simulink model "PMSM_FOC_Traction"  (R2020b)
settings: Solver=FixedStepAuto  StartTime=0.0  StopTime=10  RelTol=1e-3
model workspace (MAT data in the model file):
  wc : Simulink.Parameter (value not decoded)
values from neighbouring files (symbols this model uses):
  CL_Param = tmp_CL_Param    [PMSM_Parameters.m]
  Cosine_table = [1,0.999995293095708,0.999990587122738,0.999985881149769,0.999981174245477,0.999967055395246,0.999952936545014,0.999938818626106,0.999924698844552,0.999901168979704,0.999877639114857,0.999854108318687,0.999830577522516,0.999797635711730,0.999764694832265,0.999731753021479,0.999698810279369,0.999656459316611,0.999614108353853,0.999571758322418,0.999529405497015,0.999477646313608,0.999425887130201,0 ...(+75635 chars)    [Motor_Table.m]
  ctrlParamsPI = tmp_ctrlParamsPI    [PMSM_Parameters.m]
  Flux_weak = tmp_Fluxweak_struct    [PMSM_Parameters.m]
  FluxObsever = tmp_FluxObsever_struct    [PMSM_Parameters.m]
  Hall_Parameter = tmp_Hall_struct    [PMSM_Parameters.m]
  HFI = tmp_HFI_struct    [PMSM_Parameters.m]
  inverter = struct    [PMSM_Parameters.m]
  MTPA_id_table = [-1.39452500000000,-1.36697494250000,-1.33970177000000,-1.31270548250000,-1.28598608000000,-1.25954356250000,-1.23337793000000,-1.20748918250000,-1.18187732000000,-1.15654234250000,-1.13148425000000,-1.10670304250000,-1.08219872000000,-1.05797128250000,-1.03402073000000,-1.01034706250000,-0.986950280000000,-0.963830382500000,-0.940987370000000,-0.918421242500000,-0.896132000000000,-0.8741196425000 ...(+3439 chars)    [Motor_Table.m]
  MTPA_iq_table = [-10.2740250000000,-10.1791705677750,-10.0840783722000,-9.98875081492500,-9.89319029760000,-9.79739922187500,-9.70137998940000,-9.60513500182500,-9.50866666080000,-9.41197736797500,-9.31506952500000,-9.21794553352500,-9.12060779520000,-9.02305871167500,-8.92530068460000,-8.82733611562500,-8.72916740640000,-8.63079695857500,-8.53222717380000,-8.43346045372500,-8.33449920000000,-8.23534581427500,-8. ...(+3121 chars)    [Motor_Table.m]
  MTPA_Te_Max = single(1.50)    [Motor_Table.m]
  MTPA_Te_Min = single(-1.50)    [Motor_Table.m]
  OPL_Param = tmp_OPL_Param    [PMSM_Parameters.m]
  pmsm = struct    [PMSM_Parameters.m]
  Resolver_Parameter = tmp_Resolver_struct    [PMSM_Parameters.m]
  Sine_table = [0,0.00153398793190718,0.00306797679513693,0.00460196565836668,0.00613595545291901,0.00766988657414913,0.00920381769537926,0.0107377488166094,0.0122716808691621,0.0138054965063930,0.0153393121436238,0.0168731296434999,0.0184069443494082,0.0199405867606401,0.0214742291718721,0.0230078706517816,0.0245415139943361,0.0260749254375696,0.0276083368808031,0.0291417483240366,0.0306751597672701,0.032208281 ...(+75648 chars)    [Motor_Table.m]
  SMO = temp_SMO    [PMSM_Parameters.m]
undefined symbols (not defined in the file or in its folder): DiscIntNeverNeededParam, Kiv, Kiw, Kpv, Kpw, magnitude, sigbuilder_block, SVPWM, Vdc
libraries: powerlib x29, fl_lib x18, simulink x7, nesl_utility x7, pid_lib x5, dspstat3 x4, eeGeneralControl x4, eeDiscretePi x2, powerlib_extras x1, ee_lib x1
(part 2 of 6)

== system PMSM_FOC_Traction/PMSM/Resolver_Angle_cacl ==
  Vp_Vx_Vy : Inport
  2*pi : Constant  Value=2*pi  OutDataTypeStr=single  SampleTime=-1
  A : Selector  IndexMode=Zero-based  InputPortWidth=3  IndexOptions=Index vector (dialog)  Indices=0  OutputSizes=1
  B : Selector  IndexMode=Zero-based  InputPortWidth=3  IndexOptions=Index vector (dialog)  Indices=1  OutputSizes=1
  C : Selector  IndexMode=Zero-based  InputPortWidth=3  IndexOptions=Index vector (dialog)  Indices=2  OutputSizes=1
  Constant : Constant  Value=pmsm.PolePairs  OutDataTypeStr=single  SampleTime=-1
  Discrete-Time Integrator : DiscreteIntegrator  SampleTime=-1  ICPrevOutput=DiscIntNeverNeededParam  ICPrevScaledInput=DiscIntNeverNeededParam
  Gain : Gain  Gain=60/(2*pi)
  Math Function : Math  Operator=mod  SignedPower=on  SaturateOnIntegerOverflow=on
  PID Controller : pid_lib/PID Controller  Controller=PI  Form=Parallel  TimeDomain=Discrete-time  UseExternalTs=off  SampleTime=-1  IntegratorMethod=Forward Euler  FilterMethod=Forward Euler  ControllerParametersSource=internal  P=15  I=2.5e5  D=0  UseFilter=off  N=100  TunerSelectOption=Transfer Function Based (PID Tuner App)  InitialConditionSource=internal  InitialConditionForIntegrator=0  InitialConditionForFilter=0  DifferentiatorICPrevScaledInput=0  ExternalReset=none  TrackingMode=off  Kt=1  LimitOutput=off  SatLimitsSource=internal  UpperSaturationLimit=inf  LowerSaturationLimit=-inf  LinearizeAsGain=on  AntiWindupMode=none  Kb=1  POutMin=[]  POutMax=[]  IOutMin=[]  IOutMax=[]  DOutMin=[]  DOutMax=[]  NOutMin=[]  NOutMax=[]  SumOutMin=[]  SumOutMax=[]  SaturationOutMin=[]  SaturationOutMax=[]  PParamMin=[]  PParamMax=[]  IParamMin=[]  IParamMax=[]  DParamMin=[]  DParamMax=[]  NParamMin=[]  NParamMax=[]  KbParamMin=[]  KbParamMax=[]  KtParamMin=[]  KtParamMax=[]  KbOutMin=[]  KbOutMax=[]  KtOutMin=[]  KtOutMax=[]  IntegratorOutMin=[]  IntegratorOutMax=[]  FilterOutMin=[]  FilterOutMax=[]  SumI1OutMin=[]  SumI1OutMax=[]  SumI2OutMin=[]  SumI2OutMax=[]  SumI3OutMin=[]  SumI3OutMax=[]  SumI4OutMin=[]  SumI4OutMax=[]  SumDOutMin=[]  SumDOutMax=[]  DifferentiatorOutMin=[]  DifferentiatorOutMax=[]  FilterDiffOutCoefMin=[]  FilterDiffOutCoefMax=[]  ReciprocalOutMin=[]  ReciprocalOutMax=[]  SumDenOutMin=[]  SumDenOutMax=[]  SumNumOutMin=[]  SumNumOutMax=[]  DivideOutMin=[]  DivideOutMax=[]  UdiffTsProdOutMin=[]  UdiffTsProdOutMax=[]  NTsProdOutMin=[]  NTsProdOutMax=[]  UintegralTsProdOutMin=[]  UintegralTsProdOutMax=[]  UngainTsProdOutMin=[]  UngainTsProdOutMax=[]  IntegratorContinuousStateAttributes=''  IntegratorStateMustResolveToSignalObject=off  IntegratorRTWStateStorageClass=Auto  FilterContinuousStateAttributes=''  FilterStateMustResolveToSignalObject=off  FilterRTWStateStorageClass=Auto  ParallelPVariant=InternalParameters  IdealPVariant=Disabled  IVariant=InternalParameters  DVariant=Disabled  IntegratorVariant=Discrete  SatVariant=Disabled  AWVariant=Passthrough  PCopyVariant=Disabled  TRVariant=Disabled  FdbkBlocksVariant=Forward  IdealPFdbkVariant=Disabled  SatFdbkVariant=Disabled  DerivativeFilterVariant=Disabled  NVariant=Disabled  NCopyVariant=Disabled_SignalSpec  FilterICVariant=Disabled  IntegratorICVariant=InternalICs  ExternalResetVariant=Disabled  TRSumVariant=Passthrough  SumFdbkVariant=Disabled  SumVariant=Sum_PI  TsampFilterVariant=InternalTs  TsampNgainVariant=Passthrough  TsampIntegralVariant=Passthrough  ExternalSaturationOutDataTypeStr=Inherit: Same as second input
  Product : Product  OutDataTypeStr=single
  Product{1..4} (4 alike) : Product
  Quantizer : Quantizer  QuantizationInterval=1e-5
  Quantizer1 : Quantizer  QuantizationInterval=1e-5
  Quantizer2 : Quantizer  QuantizationInterval=1e-5
  Scope : Scope  NumInputPorts=2
  Scope{1,3..4,6} (4 alike) : Scope
  Scope2 : Scope  NumInputPorts=2
  Scope5 : Scope  NumInputPorts=2
  Sum1 : Sum  Inputs=-+
  Trigonometric Function : Trigonometry  Operator=sincos
  Unit Delay4 : UnitDelay  SampleTime=-1  HasFrameUpgradeWarning=on
  "pole pairs " : Gain  Gain=pmsm.PolePairs  OutDataTypeStr=single
  Velocity : Outport  VectorParamsAs1DForOutWhenUnconnected=off
  Angle : Outport  Port=2  VectorParamsAs1DForOutWhenUnconnected=off
  wires:
  Quantizer/1 -> Scope1/1, Product3/1
  Quantizer1/1 -> Product4/2
  Product2/1 -> Scope2/2, Product4/1
  Product4/1 -> Scope/2, Sum1/2
  Trigonometric Function/2 -> Product2/2
  Vp_Vx_Vy/1 -> C/1, B/1, A/1
  Unit Delay4/1 -> Product/2
  Sum1/1 -> PID Controller/1
  Product3/1 -> Scope/1, Sum1/1
  Constant/1 -> Product/1
  Quantizer2/1 -> Product2/1, Product1/1
  Product/1 -> Trigonometric Function/1
  Trigonometric Function/1 -> Product1/2
  Product1/1 -> Scope2/1, Product3/2
  Math Function/1 -> Angle/1, Scope4/1  "Angle1"
  Gain/1 -> Velocity/1, Scope3/1  "Speed1"
  Discrete-Time Integrator/1 -> Scope6/1, "pole pairs "/1, Unit Delay4/1
  "pole pairs "/1 -> Math Function/1
  PID Controller/1 -> Discrete-Time Integrator/1, Gain/1
  2*pi/1 -> Math Function/2
  A/1 -> Quantizer2/1  "Vp"
  B/1 -> Scope5/1, Quantizer/1, Scope5/2  "Vx"
  C/1 -> Quantizer1/1  "Vy"

== system PMSM_FOC_Traction/PMSM/Resolver_Angle_cacl1 ==
  Vp_Vx_Vy : Inport
  2*pi : Constant  Value=2*pi  OutDataTypeStr=single  SampleTime=-1
  A : Selector  IndexMode=Zero-based  InputPortWidth=3  IndexOptions=Index vector (dialog)  Indices=0  OutputSizes=1
  B : Selector  IndexMode=Zero-based  InputPortWidth=3  IndexOptions=Index vector (dialog)  Indices=1  OutputSizes=1
  C : Selector  IndexMode=Zero-based  InputPortWidth=3  IndexOptions=Index vector (dialog)  Indices=2  OutputSizes=1
  Constant : Constant  Value=pmsm.PolePairs  OutDataTypeStr=single  SampleTime=-1
  Discrete-Time Integrator : DiscreteIntegrator  SampleTime=-1  ICPrevOutput=DiscIntNeverNeededParam  ICPrevScaledInput=DiscIntNeverNeededParam
  Gain : Gain  Gain=60/(2*pi)
  LPF : DiscreteFilter  Numerator=[0 0.04]  Denominator=[1 -0.96]  SampleTime=inverter.Ts
  Math Function : Math  Operator=mod  SignedPower=on  SaturateOnIntegerOverflow=on
  PID Controller : pid_lib/PID Controller  Controller=PI  Form=Parallel  TimeDomain=Discrete-time  UseExternalTs=off  SampleTime=-1  IntegratorMethod=Forward Euler  FilterMethod=Forward Euler  ControllerParametersSource=internal  P=120  I=2500  D=0  UseFilter=off  N=100  TunerSelectOption=Transfer Function Based (PID Tuner App)  InitialConditionSource=internal  InitialConditionForIntegrator=0  InitialConditionForFilter=0  DifferentiatorICPrevScaledInput=0  ExternalReset=none  TrackingMode=off  Kt=1  LimitOutput=off  SatLimitsSource=internal  UpperSaturationLimit=inf  LowerSaturationLimit=-inf  LinearizeAsGain=on  AntiWindupMode=none  Kb=1  POutMin=[]  POutMax=[]  IOutMin=[]  IOutMax=[]  DOutMin=[]  DOutMax=[]  NOutMin=[]  NOutMax=[]  SumOutMin=[]  SumOutMax=[]  SaturationOutMin=[]  SaturationOutMax=[]  PParamMin=[]  PParamMax=[]  IParamMin=[]  IParamMax=[]  DParamMin=[]  DParamMax=[]  NParamMin=[]  NParamMax=[]  KbParamMin=[]  KbParamMax=[]  KtParamMin=[]  KtParamMax=[]  KbOutMin=[]  KbOutMax=[]  KtOutMin=[]  KtOutMax=[]  IntegratorOutMin=[]  IntegratorOutMax=[]  FilterOutMin=[]  FilterOutMax=[]  SumI1OutMin=[]  SumI1OutMax=[]  SumI2OutMin=[]  SumI2OutMax=[]  SumI3OutMin=[]  SumI3OutMax=[]  SumI4OutMin=[]  SumI4OutMax=[]  SumDOutMin=[]  SumDOutMax=[]  DifferentiatorOutMin=[]  DifferentiatorOutMax=[]  FilterDiffOutCoefMin=[]  FilterDiffOutCoefMax=[]  ReciprocalOutMin=[]  ReciprocalOutMax=[]  SumDenOutMin=[]  SumDenOutMax=[]  SumNumOutMin=[]  SumNumOutMax=[]  DivideOutMin=[]  DivideOutMax=[]  UdiffTsProdOutMin=[]  UdiffTsProdOutMax=[]  NTsProdOutMin=[]  NTsProdOutMax=[]  UintegralTsProdOutMin=[]  UintegralTsProdOutMax=[]  UngainTsProdOutMin=[]  UngainTsProdOutMax=[]  IntegratorContinuousStateAttributes=''  IntegratorStateMustResolveToSignalObject=off  IntegratorRTWStateStorageClass=Auto  FilterContinuousStateAttributes=''  FilterStateMustResolveToSignalObject=off  FilterRTWStateStorageClass=Auto  ParallelPVariant=InternalParameters  IdealPVariant=Disabled  IVariant=InternalParameters  DVariant=Disabled  IntegratorVariant=Discrete  SatVariant=Disabled  AWVariant=Passthrough  PCopyVariant=Disabled  TRVariant=Disabled  FdbkBlocksVariant=Forward  IdealPFdbkVariant=Disabled  SatFdbkVariant=Disabled  DerivativeFilterVariant=Disabled  NVariant=Disabled  NCopyVariant=Disabled_SignalSpec  FilterICVariant=Disabled  IntegratorICVariant=InternalICs  ExternalResetVariant=Disabled  TRSumVariant=Passthrough  SumFdbkVariant=Disabled  SumVariant=Sum_PI  TsampFilterVariant=InternalTs  TsampNgainVariant=Passthrough  TsampIntegralVariant=Passthrough  ExternalSaturationOutDataTypeStr=Inherit: Same as second input
  Product : Product  OutDataTypeStr=single
  Product{1..4} (4 alike) : Product
  Quantizer : Quantizer  QuantizationInterval=1e-5
  Quantizer1 : Quantizer  QuantizationInterval=1e-5
  Quantizer2 : Quantizer  QuantizationInterval=1e-5
  Scope : Scope  NumInputPorts=2
  Scope{1,3..4,6} (4 alike) : Scope
  Scope2 : Scope  NumInputPorts=2
  Scope5 : Scope  NumInputPorts=2
  Sum1 : Sum  Inputs=-+
  Trigonometric Function : Trigonometry  Operator=sincos
  Unit Delay4 : UnitDelay  SampleTime=-1  HasFrameUpgradeWarning=on
  "pole pairs " : Gain  Gain=pmsm.PolePairs  OutDataTypeStr=single
  Velocity : Outport  VectorParamsAs1DForOutWhenUnconnected=off
  Angle : Outport  Port=2  VectorParamsAs1DForOutWhenUnconnected=off
  wires:
  Quantizer/1 -> Scope1/1, Product3/1, Scope5/2
  Quantizer1/1 -> Product4/2
  Product2/1 -> Scope2/2, Product4/1
  Product4/1 -> Scope/2, Sum1/2
  Trigonometric Function/2 -> Product2/2
  Vp_Vx_Vy/1 -> C/1, B/1, A/1
  Unit Delay4/1 -> Product/2
  Sum1/1 -> PID Controller/1
  Product3/1 -> Scope/1, Sum1/1
  Constant/1 -> Product/1
  Quantizer2/1 -> Product2/1, Product1/1
  Product/1 -> Trigonometric Function/1
  Trigonometric Function/1 -> Product1/2
  Product1/1 -> Scope2/1, Product3/2
  Math Function/1 -> Angle/1, Scope4/1  "Angle"
  Gain/1 -> LPF/1, Scope3/1  "Speed"
  Discrete-Time Integrator/1 -> Scope6/1, "pole pairs "/1, Unit Delay4/1
  "pole pairs "/1 -> Math Function/1
  PID Controller/1 -> Discrete-Time Integrator/1, Gain/1
  2*pi/1 -> Math Function/2
  A/1 -> Quantizer2/1  "Vp"
  B/1 -> Scope5/1, Quantizer/1  "Vx"
  C/1 -> Quantizer1/1  "Vy"
  LPF/1 -> Velocity/1

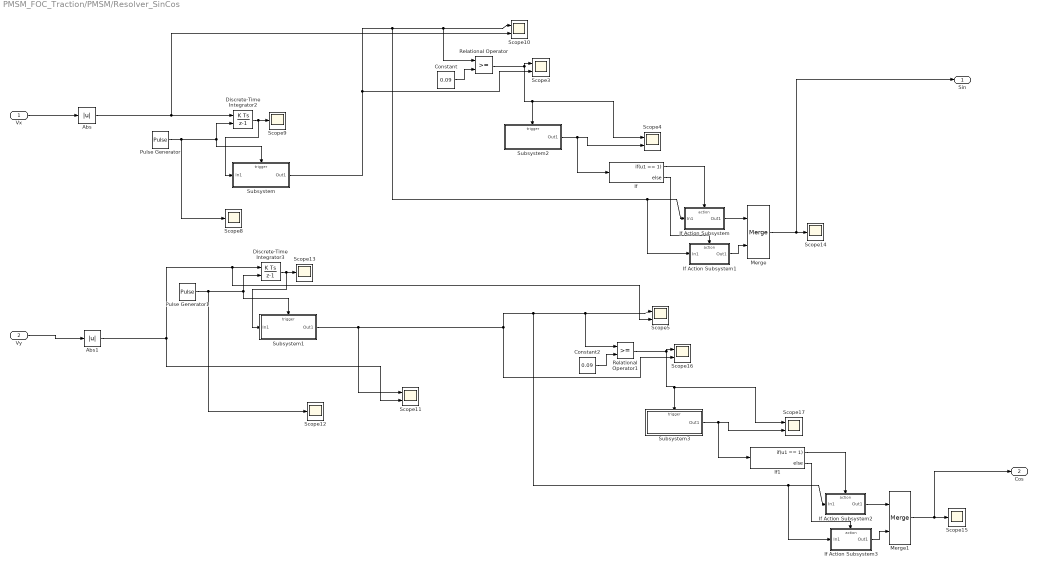
== system PMSM_FOC_Traction/PMSM/Resolver_SinCos ==
  Vx : Inport
  Vy : Inport  Port=2
  Abs : Abs
  Abs1 : Abs
  Constant : Constant  Value=0.09
  Constant2 : Constant  Value=0.09
  Discrete-Time Integrator2 : DiscreteIntegrator  gainval=15625  ExternalReset=falling  SampleTime=-1  ICPrevOutput=DiscIntNeverNeededParam  ICPrevScaledInput=DiscIntNeverNeededParam
  Discrete-Time Integrator3 : DiscreteIntegrator  gainval=15625  ExternalReset=falling  SampleTime=-1  ICPrevOutput=DiscIntNeverNeededParam  ICPrevScaledInput=DiscIntNeverNeededParam
  If : If  IfExpression=u1 == 1
  If Action Subsystem : Subsystem  TreatAsAtomicUnit=on
  If Action Subsystem1 : Subsystem  TreatAsAtomicUnit=on
  If Action Subsystem2 : Subsystem  TreatAsAtomicUnit=on
  If Action Subsystem3 : Subsystem  TreatAsAtomicUnit=on
  If1 : If  IfExpression=u1 == 1
  Merge : Merge
  Merge1 : Merge
  Pulse Generator : DiscretePulseGenerator  PulseType=Time based  Period=inverter.Ts  PulseWidth=5
  Pulse Generator1 : DiscretePulseGenerator  PulseType=Time based  Period=inverter.Ts  PulseWidth=5
  Relational Operator : RelationalOperator  OutDataTypeStr=boolean  RndMeth=Simplest
  Relational Operator1 : RelationalOperator  OutDataTypeStr=boolean  RndMeth=Simplest
  Scope{3..5,10..11,16..17} (7 alike) : Scope  NumInputPorts=2
  Scope{8..9,12..15} (6 alike) : Scope
  Subsystem : Subsystem
  Subsystem1 : Subsystem
  Subsystem2 : Subsystem
  Subsystem3 : Subsystem
  Sin : Outport
  Cos : Outport  Port=2
  wires:
  Discrete-Time Integrator2/1 -> Subsystem/1(In1), Scope9/1
  Subsystem/1(Out1) -> If Action Subsystem1/1(In1), If Action Subsystem/1(In1), Relational Operator/1, Scope10/1, Scope3/2
  Subsystem2/1(Out1) -> If/1, Scope4/2
  Pulse Generator/1 -> Scope8/1, Discrete-Time Integrator2/2, Subsystem/Trigger
  If Action Subsystem2/1(Out1) -> Merge1/1
  If1/1 -> If Action Subsystem2/Action
  Relational Operator1/1 -> Scope17/1, Subsystem3/Trigger, Scope16/1
  Merge1/1 -> Cos/1, Scope15/1
  Constant2/1 -> Relational Operator1/2
  Subsystem3/1(Out1) -> If1/1, Scope17/2
  Abs1/1 -> Scope5/2, Discrete-Time Integrator3/1, Scope11/2
  If/2 -> If Action Subsystem1/Action
  Constant/1 -> Relational Operator/2
  If1/2 -> If Action Subsystem3/Action
  Relational Operator/1 -> Scope4/1, Subsystem2/Trigger, Scope3/1
  Pulse Generator1/1 -> Scope12/1, Discrete-Time Integrator3/2, Subsystem1/Trigger
  Abs/1 -> Scope10/2, Discrete-Time Integrator2/1
  Discrete-Time Integrator3/1 -> Subsystem1/1(In1), Scope13/1
  Merge/1 -> Sin/1, Scope14/1
  If Action Subsystem1/1(Out1) -> Merge/2
  Subsystem1/1(Out1) -> If Action Subsystem3/1(In1), If Action Subsystem2/1(In1), Relational Operator1/1, Scope5/1, Scope16/2, Scope11/1
  If Action Subsystem/1(Out1) -> Merge/1
  If Action Subsystem3/1(Out1) -> Merge1/2
  If/1 -> If Action Subsystem/Action
  Vx/1 -> Abs/1
  Vy/1 -> Abs1/1

== system PMSM_FOC_Traction/PMSM/SVPWM2 ==
  Gate : Inport
  Duty : Inport  Port=2
  Add{1..6} (6 alike) : Sum  Inputs=+-
  Bus Creator : BusCreator  Inputs=6
  Demux1 : Demux  Outputs=6
  Gain2 : Gain  Gain=4200
  Product{1..6} (6 alike) : Product
  Relay{,1..5} (6 alike) : Relay  OnOutputValue=0  OffOutputValue=1
  Repeating Sequence2 : simulink/Sources/Repeating Sequence  rep_seq_t=[0 inverter.Ts/2 inverter.Ts]  rep_seq_y=[0 4200 0]
  Scope : Scope  NumInputPorts=2
  Scope1 : Scope  NumInputPorts=2
  pulse : Outport
  wires:
  Repeating Sequence2/1 -> Add1/1, Add4/1, Add2/1, Add5/1, Add6/1, Add3/1
  Product2/1 -> Add2/2
  Product3/1 -> Add3/2
  Add3/1 -> Relay2/1
  Add2/1 -> Relay1/1
  Add1/1 -> Relay/1
  Product1/1 -> Add1/2
  Bus Creator/1 -> pulse/1
  Gate/1 -> Demux1/1
  Demux1/1 -> Product1/1, Scope/1
  Demux1/3 -> Product2/1
  Demux1/5 -> Product3/1
  Gain2/1 -> Product4/2, Product1/2, Product5/2, Product6/2, Product3/2, Product2/2
  Demux1/2 -> Product4/1
  Demux1/4 -> Product5/1
  Demux1/6 -> Scope1/2, Product6/1
  Add4/1 -> Relay3/1
  Add5/1 -> Relay4/1
  Add6/1 -> Relay5/1
  Product6/1 -> Add6/2
  Product5/1 -> Add5/2
  Product4/1 -> Add4/2
  Relay/1 -> Scope/2, Bus Creator/1
  Relay3/1 -> Bus Creator/2
  Relay1/1 -> Bus Creator/3
  Relay2/1 -> Bus Creator/5
  Relay5/1 -> Bus Creator/6, Scope1/1
  Duty/1 -> Gain2/1
  Relay4/1 -> Bus Creator/4

== system PMSM_FOC_Traction/PMSM/SpeedAndAngle ==
  Hall : Inport
  Counter : Inport  Port=2
  ACC_OMG : Subsystem  TreatAsAtomicUnit=on
      settings: RTWSystemCode=Nonreusable function  RTWFcnNameOpts=Use subsystem name
  ADC_IRQ : Subsystem  TreatAsAtomicUnit=on
      settings: RTWSystemCode=Nonreusable function  RTWFcnNameOpts=Use subsystem name
  Demux : Demux  Outputs=3
  Scope : Scope
  Hall_Angle : Outport
  Hall_Speed_RPM : Outport  Port=2
  Six_theta : Outport  Port=3
  wires:
  Demux/2 -> ACC_OMG/3(HallB)
  Demux/3 -> ACC_OMG/4(HallC)
  ACC_OMG/1(Hall_SpeedRPM) -> Hall_Speed_RPM/1
  Counter/1 -> ACC_OMG/1(Timer_Counter), ADC_IRQ/1(Counter_ADC_IRQ)
  Demux/1 -> ACC_OMG/2(HallA)
  ACC_OMG/5(Six_theta) -> ADC_IRQ/5(Six_theta)
  ACC_OMG/2(Acc) -> ADC_IRQ/2(Acc)
  ACC_OMG/3(OMG) -> ADC_IRQ/3(OMG)
  Hall/1 -> ACC_OMG/Trigger, Demux/1
  ACC_OMG/4(Counter) -> ADC_IRQ/4(Counter_Hall_IRQ)
  ADC_IRQ/1(Hall_Angle) -> Hall_Angle/1, Scope/1
  ACC_OMG/6(Six_theta1) -> Six_theta/1

== system PMSM_FOC_Traction/PMSM/Timer_Counter ==
  Add2 : Sum
  Constant3 : Constant  OutDataTypeStr=single
  Memory : Memory  InheritSampleTime=on
  Counter : Outport
  wires:
  Add2/1 -> Counter/1, Memory/1
  Constant3/1 -> Add2/1
  Memory/1 -> Add2/2

== system PMSM_FOC_Traction/PMSM/Timer_Counter1 ==
  Add2 : Sum
  Constant3 : Constant  OutDataTypeStr=single
  Memory : Memory  InheritSampleTime=on
  Counter : Outport
  wires:
  Add2/1 -> Counter/1, Memory/1
  Constant3/1 -> Add2/1
  Memory/1 -> Add2/2

== system PMSM_FOC_Traction/PMSM/W_R ==
  w : Inport
  Angular Velocity Source : fl_lib/Mechanical/Mechanical Sources/Ideal Angular Velocity Source
  Mechanical Rotational Reference2 : fl_lib/Mechanical/Rotational Elements/Mechanical Rotational Reference
  Simulink-PS Converter : nesl_utility/Simulink-PS Converter  PhysicalDomain=network_engine_domain  SubClassName=ps_input  LeftPortType=input  RightPortType=output  PseudoPeriodic=off  Frequencies=[]  NoiseDistribution=none  NoiseParameters=[]  Unit=rad/s  AffineConversion=off  FilteringAndDerivatives=zero  SimscapeFilterOrder=1  InputFilterTimeConstant=0.0001  UdotUserProvided=1
  Torque Sensor : Subsystem
  R : PMIOPort  Side=Right
  C : PMIOPort  Port=2  Side=Right
  tag scope: wref=global
  wires:
  w/1 -> [wref], Simulink-PS Converter/1
  connections:
  Mechanical Rotational Reference2/LConn1 -- C/RConn1 -- Angular Velocity Source/RConn2
  Simulink-PS Converter/RConn1 -- Angular Velocity Source/RConn1
  Torque Sensor/LConn1 -- R/RConn1
  Torque Sensor/RConn1 -- Angular Velocity Source/LConn1

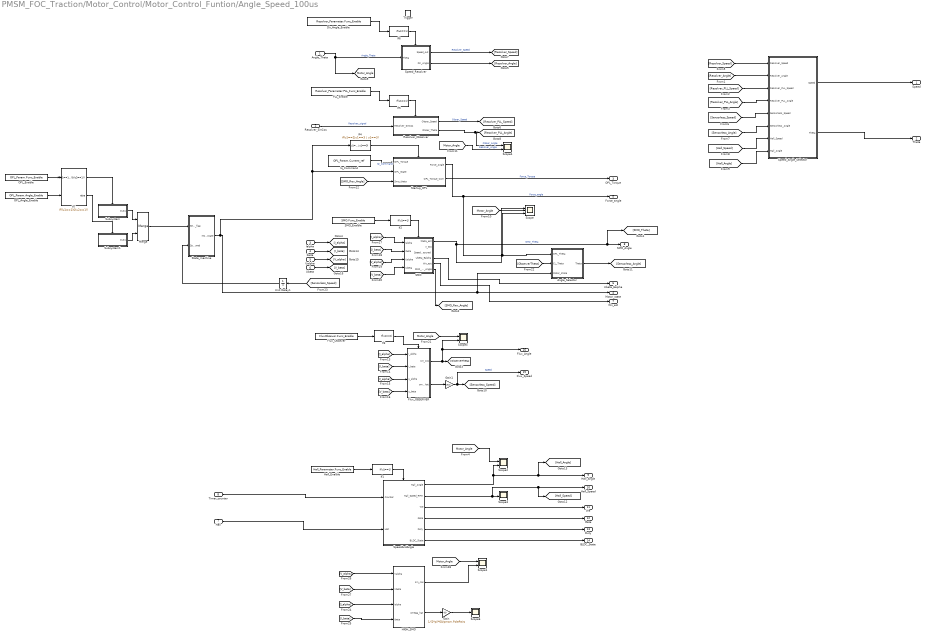
== system PMSM_FOC_Traction/Motor_Control/Motor_Control_Funtion/Angle_Speed_100us ==
  Angle_Theta : Inport  OutMin=0  OutMax=2*pi
  Resolver_SinCos : Inport  Port=2  OutMin=0  OutMax=2*pi
  Ialpha : Inport  Port=3
  Ibeta : Inport  Port=4
  Ualpha : Inport  Port=5
  Ubeta : Inport  Port=6
  Hall : Inport  Port=7
  Timer_counter : Inport  Port=8
  Trigger : TriggerPort  TriggerType=function-call  VariantControl=Variant  SampleTimeType=periodic  SampleTime=-1  PortDimensions=1
  Angle_Selector : Subsystem  TreatAsAtomicUnit=on
      settings: RTWSystemCode=Nonreusable function  RTWFcnNameOpts=Use subsystem name
  Dir_Angle_Enable : Constant  Value=Resolver_Parameter.Func_Enable  OutDataTypeStr=uint8
  Flux_OBSERVER : Subsystem
  Flux_Obsever : Constant  Value=FluxObsever.Func_Enable  OutDataTypeStr=uint8
  Gain : Gain  Gain=1/(2*pi)*60/pmsm.PolePairs
  Gain1 : Gain  Gain=15/pi  OutDataTypeStr=Inherit: Same as input  ParamDataTypeStr=Inherit: Same as input
  HIGH_SMO : Subsystem
      mask Display:
      | port_label('input',1,'U_\alpha','texmode','on');
      | port_label('input',2,'U_\beta','texmode','on');
      | port_label('input',3,'I_\alpha','texmode','on');
      | port_label('input',4,'I_\beta','texmode','on');
      | 
      | port_label('output',1,'sin(\theta_e)cos(\theta_e)','texmode','on');
      | port_label('output',2,'\omega_e','texmode','on');
      | 
      | fprintf('HSMO');
  Hall_Enalble : Constant  Value=Hall_Parameter.Func_Enable  OutDataTypeStr=uint8
  If{1..3,5..6} (5 alike) : If  IfExpression=u1==1  ShowElse=off
  If4 : If  IfExpression=u1==2|u1==3 | u1==3  ShowElse=off
  If7 : If  NumInputs=2  IfExpression=(u1==1)&(u2==1)
  Iq_Command : Constant  Value=OPL_Param.Current_ref  SampleTime=-1
  Merge : Merge
  OPL_Angle_Enable : Constant  Value=OPL_Param.Angle_Enable  OutDataTypeStr=uint8
  OPL_Enable : Constant  Value=OPL_Param.Func_Enable  OutDataTypeStr=uint8
  PLL_Enable : Constant  Value=Resolver_Parameter.PLL_Func_Enable  OutDataTypeStr=uint8
  Resolver_Observer : Subsystem
      settings: RTWSystemCode=Nonreusable function  RTWFcnNameOpts=Use subsystem name
  SMO : Subsystem  TreatAsAtomicUnit=on
      settings: RTWSystemCode=Nonreusable function  RTWFcnNameOpts=Use subsystem name
  SMO_Enalble : Constant  Value=SMO.Func_Enable  OutDataTypeStr=uint8
  Scope : Scope  NumInputPorts=3
  Scope{1..2,4..5} (4 alike) : Scope  NumInputPorts=2
  Scope3 : Scope
  Scope6 : Scope
  SpeedAndAngle : Subsystem
      settings: RTWSystemCode=Nonreusable function  RTWFcnNameOpts=Use subsystem name  RTWFileNameOpts=Use subsystem name
  Speed_Angle_Selector : Subsystem
  Speed_Resolver : Subsystem  TreatAsAtomicUnit=on
      settings: RTWSystemCode=Nonreusable function  RTWFcnNameOpts=Use subsystem name
  Startup_OPL : Subsystem  TreatAsAtomicUnit=on  SystemSampleTime=inverter.Ts
      settings: RTWSystemCode=Nonreusable function  RTWFcnNameOpts=Use subsystem name
  State_machine : Stateflow chart  TreatAsAtomicUnit=on
      settings: RTWSystemCode=Nonreusable function  RTWFcnNameOpts=Use subsystem name
  Subsystem : Subsystem
  Subsystem1 : Subsystem
  Unit Delay1 : UnitDelay  SampleTime=-1  HasFrameUpgradeWarning=on
  Speed : Outport
  Theta : Outport  Port=2
  OPL_Torque : Outport  Port=3
  Motor_state : Outport  Port=4
  Force_angle : Outport  Port=5
  Ubeta_Ealpha : Outport  Port=6
  Wn_est : Outport  Port=7
  SMO_Angle : Outport  Port=8
  Hall_Angle : Outport  Port=9
  Hall_Speed : Outport  Port=10
  We : Outport  Port=11
  Gate : Outport  Port=12  VectorParamsAs1DForOutWhenUnconnected=off
  Duty : Outport  Port=13  VectorParamsAs1DForOutWhenUnconnected=off
  BLDC_State : Outport  Port=14  VectorParamsAs1DForOutWhenUnconnected=off
  Flux_Speed : Outport  Port=15
  Flux_Angle : Outport  Port=16
  tag scope: Motor_Angle=global
  wires:
  Resolver_SinCos/1 -> Resolver_Observer/1(Resolver_SinCos)  "Resolver_signal"
  Iq_Command/1 -> Startup_OPL/1(OPL_Torque)  "IQ_Command"
  Resolver_Observer/2(Obser_Theta) -> Scope4/1, [Resolver_PLL_Angle]  "Obser_Angle"
  Ialpha/1 -> [I_alpha]
  Speed_Resolver/1(Speed_out) -> [Resolver_Speed]  "Resolver_Speed"
  Angle_Theta/1 -> [Motor_Angle], Speed_Resolver/1(Theta)  "Angle_Theta"
  Resolver_Observer/1(Obser_Speed) -> [Resolver_PLL_Speed]  "Obser_Speed"
  Startup_OPL/2(OPL_Torque_Com) -> OPL_Torque/1  "Force_Torque"
  Speed_Resolver/2(Dir_Angle) -> [Resolver_Angle]
  State_machine/1(Motor_state) -> Startup_OPL/2(OPL_State), If4/1, Angle_Selector/3(Motor_state), Motor_state/1
  Unit Delay1/1 -> State_machine/2(Speed_Measured)
  SMO/1(theta_est) -> Scope/1, [SMO_Theta], SMO_Angle/1  "SMO_Theta"
  Startup_OPL/1(Force_Angle) -> Scope/3, Angle_Selector/1(OPL_Theta), Force_angle/1  "Force_angle"
  Angle_Selector/1(Theta) -> [Sensorless_Angle]
  [Motor_Angle] -> Scope2/1
  SMO/4(Ubeta_Ealpha) -> Ubeta_Ealpha/1
  SMO/5(Wn_est) -> Wn_est/1
  Hall/1 -> SpeedAndAngle/2(Hall)
  Timer_counter/1 -> SpeedAndAngle/1(Counter)
  SpeedAndAngle/1(Hall_Angle) -> Scope2/2, Hall_Angle/1, [Hall_Angle]
  SpeedAndAngle/2(Hall_Speed_RPM) -> Hall_Speed/1, [Hall_Speed], Scope3/1
  If1/1 -> SpeedAndAngle/Action
  Hall_Enalble/1 -> If1/1
  SMO_Enalble/1 -> If2/1
  PLL_Enable/1 -> If5/1
  If5/1 -> Resolver_Observer/Action
  If6/1 -> Speed_Resolver/Action
  Dir_Angle_Enable/1 -> If6/1
  If4/1 -> Startup_OPL/Action
  [Resolver_Speed] -> Speed_Angle_Selector/1(Resolver_Speed)
  [Resolver_Angle] -> Speed_Angle_Selector/2(Resolver_Angle)
  [Resolver_PLL_Speed] -> Speed_Angle_Selector/3(Resolver_PLL_Speed)
  [Resolver_PLL_Angle] -> Speed_Angle_Selector/4(Resolver_PLL_Angle)
  [Sensorless_Speed] -> Speed_Angle_Selector/5(Sensorless_Speed)
  [Sensorless_Angle] -> Speed_Angle_Selector/6(Sensorless_Angle)
  [Hall_Speed] -> Speed_Angle_Selector/7(Hall_Speed)
  [Hall_Angle] -> Speed_Angle_Selector/8(Hall_Angle)
  [Motor_Angle] -> Scope/2
  [Motor_Angle] -> Scope4/2  "Resolver_Angle"
  OPL_Enable/1 -> If7/1
  OPL_Angle_Enable/1 -> If7/2
  If7/1 -> Subsystem/Action
  If7/2 -> Subsystem1/Action
  Subsystem/1(Out1) -> Merge/1
  Subsystem1/1(Out1) -> Merge/2
  Merge/1 -> State_machine/1(Sensorless_flag)
  [SMO_Rev_Angle] -> Startup_OPL/3(Smo_theta)
  SMO/6(SMO_Rev_Angle) -> [SMO_Rev_Angle]
  SpeedAndAngle/3(We) -> We/1
  SpeedAndAngle/5(Duty) -> Duty/1
  SpeedAndAngle/4(Gate) -> Gate/1
  SpeedAndAngle/6(BLDC_State) -> BLDC_State/1
  Speed_Angle_Selector/1(Speed) -> Speed/1
  Speed_Angle_Selector/2(Theta) -> Theta/1
  [I_beta] -> Flux_OBSERVER/2(i_beta)
  [I_alpha] -> Flux_OBSERVER/1(i_alpha)
  [V_alpha] -> Flux_OBSERVER/3(u_alpha)
  [V_beta] -> Flux_OBSERVER/4(u_beta)
  Flux_OBSERVER/1(sin_cos) -> Scope5/2, Flux_Angle/1, [ObserverTheta]
  Ibeta/1 -> [I_beta]
  Ualpha/1 -> [V_alpha]
  Ubeta/1 -> [V_beta]
  [V_alpha] -> SMO/3(Ualpha)
  [I_alpha] -> SMO/1(Ialpha)
  [I_beta] -> SMO/2(Ibeta)
  [V_beta] -> SMO/4(Ubeta)
  [Motor_Angle] -> Scope5/1
  If2/1 -> SMO/Action
  Flux_Obsever/1 -> If3/1
  If3/1 -> Flux_OBSERVER/Action
  [ObserverTheta] -> Angle_Selector/2(CL_Theta)
  Flux_OBSERVER/2(omega_e_hat) -> Gain1/1
  Gain1/1 -> Flux_Speed/1, [Sensorless_Speed]  "Speed"
  [Sensorless_Speed] -> Unit Delay1/1
  [V_alpha] -> HIGH_SMO/1(Valpha)
  [V_beta] -> HIGH_SMO/2(Vbeta)
  [I_alpha] -> HIGH_SMO/3(Ialpha)
  [I_beta] -> HIGH_SMO/4(Ibeta)
  [Motor_Angle] -> Scope1/1
  HIGH_SMO/1(sin_cos) -> Scope1/2
  HIGH_SMO/2(omega_hat) -> Gain/1
  Gain/1 -> Scope6/1

== system PMSM_FOC_Traction/Motor_Control/Motor_Control_Funtion/Control_Command_2ms ==
  Control_Mode : Inport
  Speed_target : Inport  Port=2
  Speed_Mesured : Inport  Port=3  OutMin=0  OutMax=2*pi
  HFI_State : Inport  Port=4
  Motor_State : Inport  Port=5
  BLDC_State : Inport  Port=6
  Trigger : TriggerPort  TriggerType=function-call  VariantControl=Variant  SampleTimeType=periodic  SampleTime=-1  PortDimensions=1
  IQ_Command : Constant  Value=CL_Param.Current_IQref  OutDataTypeStr=single  SampleTime=-1
  Merge : Merge
  Speed_PI : Subsystem  TreatAsAtomicUnit=on  SystemSampleTime=inverter.Ts
      settings: RTWSystemCode=Nonreusable function
  Switch Case : SwitchCase  CaseConditions={1,2}
  Switch Case Action Subsystem : Subsystem  TreatAsAtomicUnit=on
      settings: RTWSystemCode=Nonreusable function
  Te_ref : Outport
  wires:
  Switch Case Action Subsystem/1(Iq_out) -> Merge/2
  IQ_Command/1 -> Switch Case Action Subsystem/1(Iq_in)  "IQ_Command"
  Switch Case/3 -> [default]
  [Torque_Mode] -> Switch Case Action Subsystem/Action
  Switch Case/2 -> [Torque_Mode]
  Switch Case/1 -> [Speed_Mode]
  Control_Mode/1 -> Switch Case/1  "Control_ModeCommand"
  [Speed_Mode] -> Speed_PI/Action
  Speed_PI/1(Iq_ref) -> Merge/1  "Iq_ref"
  Merge/1 -> Te_ref/1
  Speed_target/1 -> Speed_PI/1(Speed_Command)  "Speed_target"
  Speed_Mesured/1 -> Speed_PI/2(Speed_Measured)  "Speed_Measured"
  HFI_State/1 -> Speed_PI/3(HFI_State)
  Motor_State/1 -> Speed_PI/4(Motor_State)
  BLDC_State/1 -> Speed_PI/5(BLDC_State)

== system PMSM_FOC_Traction/Motor_Control/Motor_Control_Funtion/FOC_Control_100us ==
  Phase_CurrentABC : Inport  PortDimensions=3
  Angle_Theta : Inport  Port=2  OutMin=0  OutMax=2*pi
  Te_ref : Inport  Port=3
  Motor_state : Inport  Port=4
  OPL_Iq : Inport  Port=5
  BLDC_State : Inport  Port=6
  Trigger : TriggerPort  TriggerType=function-call  VariantControl=Variant  SampleTimeType=periodic  SampleTime=-1  PortDimensions=1
  FOC : Subsystem  TreatAsAtomicUnit=on
      settings: RTWSystemCode=Nonreusable function  RTWFcnNameOpts=Use subsystem name
  Hall_Enalble : Constant  Value=Hall_Parameter.BLDC_Start  OutDataTypeStr=uint8
  If1 : If  NumInputs=2  IfExpression=(u1==1)&(u2==3)|(u1~=1)  ShowElse=off
  Iq_selector : Subsystem  TreatAsAtomicUnit=on
      settings: RTWSystemCode=Nonreusable function  RTWFcnNameOpts=Use subsystem name
  MTPA : Subsystem  TreatAsAtomicUnit=on
      settings: RTWSystemCode=Nonreusable function  RTWFcnNameOpts=Use subsystem name
  Ta : Outport
  Tb : Outport  Port=2
  Tc : Outport  Port=3
  Ialpha : Outport  Port=4
  Ibeta : Outport  Port=5
  Valpha : Outport  Port=6
  Vbeta : Outport  Port=7
  Id : Outport  Port=8
  Iq : Outport  Port=9
  HFI_Theta : Outport  Port=10
  RUN_State : Outport  Port=11
  HFI_Speed : Outport  Port=12
  Vd : Outport  Port=13
  Vq : Outport  Port=14
  wires:
  FOC/1(Ta) -> Ta/1  "Ta"
  FOC/2(Tb) -> Tb/1  "Tb"
  FOC/3(Tc) -> Tc/1  "Tc"
  Angle_Theta/1 -> FOC/3(Angle_Theta)  "Angle_Theta"
  FOC/4(Ialpha) -> Ialpha/1  "Ialpha"
  FOC/5(Ibeta) -> Ibeta/1  "Ibeta"
  FOC/6(Valpha) -> Valpha/1  "V_alpha"
  FOC/7(Vbeta) -> Vbeta/1  "V_beta"
  FOC/8(Id) -> Id/1  "Id_measured"
  FOC/9(Iq) -> Iq/1  "Iq_measured"
  Phase_CurrentABC/1 -> FOC/4(Phase_CurrentABC)  "Phase_CurrentABC"
  FOC/13(HFI_Theta) -> HFI_Theta/1  "HFI_Theta"
  FOC/12(RUN_State) -> RUN_State/1
  FOC/14(HFI_Speed) -> HFI_Speed/1
  MTPA/1(Id_ref) -> FOC/1(Id_target)  "Id_ref"
  MTPA/2(Iq_ref) -> Iq_selector/2(PI_IQ)  "Iq_ref"
  Iq_selector/1(Iq_ref) -> FOC/2(Iq_target)
  Te_ref/1 -> MTPA/1(Te_ref)
  Motor_state/1 -> Iq_selector/1(Motor_state)
  OPL_Iq/1 -> Iq_selector/3(OPL_IQ)
  FOC/11(Vq) -> Vq/1
  FOC/10(Vd) -> Vd/1
  Hall_Enalble/1 -> If1/1
  BLDC_State/1 -> If1/2
  If1/1 -> FOC/Action

== system PMSM_FOC_Traction/Motor_Control/Motor_Control_Funtion/Motor_State_10ms ==
  Id : Inport
  Vd : Inport  Port=2
  Iq : Inport  Port=3
  Vq : Inport  Port=4
  Trigger : TriggerPort  TriggerType=function-call  VariantControl=Variant  SampleTimeType=periodic  SampleTime=-1  PortDimensions=1
  Low pass filter : DiscreteTransferFcn  Numerator=[1-exp(-2*pi*20*inverter.Ts)]  Denominator=[1 -exp(-2*pi*20*inverter.Ts)]
  Low pass filter1 : DiscreteTransferFcn  Numerator=[1-exp(-2*pi*20*inverter.Ts)]  Denominator=[1 -exp(-2*pi*20*inverter.Ts)]
  Power_Cacl : Subsystem
  Scope{1..4} (4 alike) : Scope
  Torque_Cacl : Subsystem
  Motor_Power : Outport
  Torque : Outport  Port=2
  wires:
  Iq/1 -> Torque_Cacl/2(Iq), Power_Cacl/3(Iq)
  Low pass filter1/1 -> Torque/1, Scope4/1
  Vq/1 -> Power_Cacl/4(Vq)
  Power_Cacl/1(Power) -> Scope1/1, Low pass filter/1  "Motor_Power"
  Vd/1 -> Power_Cacl/2(Vd)
  Id/1 -> Torque_Cacl/1(Id), Power_Cacl/1(Id)
  Torque_Cacl/1(Torque) -> Low pass filter1/1, Scope2/1  "Te"
  Low pass filter/1 -> Scope3/1, Motor_Power/1

== system PMSM_FOC_Traction/PMSM/Commutation/Bit concatenate ==
  u : Inport
  Gain : Gain  Gain=[4 2 1]  Multiplication=Matrix(K*u)
  Sum of Elements : Sum  Inputs=+
  y : Outport  VectorParamsAs1DForOutWhenUnconnected=off
  wires:
  u/1 -> Gain/1
  Gain/1 -> Sum of Elements/1
  Sum of Elements/1 -> y/1

== system PMSM_FOC_Traction/PMSM/Commutation1/Bit concatenate ==
  u : Inport
  Gain : Gain  Gain=[4 2 1]  Multiplication=Matrix(K*u)
  Sum of Elements : Sum  Inputs=+
  y : Outport  VectorParamsAs1DForOutWhenUnconnected=off
  wires:
  u/1 -> Gain/1
  Gain/1 -> Sum of Elements/1
  Sum of Elements/1 -> y/1

== system PMSM_FOC_Traction/PMSM/Control/Control ==
  RPMReq : Inport
  w_sens : Inport  Port=2
  Hall : Inport  Port=3
  Vdc : Inport  Port=4
  Commutation : Subsystem
  Constant : Constant  Value=0  SampleTime=-1
  Constant1 : Constant  Value=0  SampleTime=inverter.Ts
  Rate Transition1 : RateTransition
  Rate Transition2 : RateTransition
  Rate Transition3 : RateTransition  OutPortSampleTime=inverter.Ts
  Rate Transition4 : RateTransition  OutPortSampleTime=inverter.Ts
  Rate Transition6 : RateTransition
  Speed controller : eeDiscretePi/Discrete PI Controller with Integral Anti-Windup  Kp=Kpw  Ki=Kiw  x0=0  B=Vdc  A=0  Ts=inverter.Ts
      settings: SourceProductBaseCode=PS
  Sum : Sum  Inputs=|+-
  Sum1 : Sum  Inputs=|+-
  Vdc filter : eeGeneralControl/Low-Pass Filter (Discrete or Continuous)  K=1  T=0.01  B=inf  A=-inf  init_option=Inherited from block input  x0=0  Ts=inverter.Ts
  Voltage controller : eeDiscretePi/Discrete PI Controller with Integral Anti-Windup  Kp=Kpv  Ki=Kiv  x0=0  B=1  A=0  Ts=inverter.Ts
      settings: SourceProductBaseCode=PS
  rad/s->rpm : Gain  Gain=30/pi
  S : Outport  VectorParamsAs1DForOutWhenUnconnected=off
  Duty : Outport  Port=2  VectorParamsAs1DForOutWhenUnconnected=off
  tag scope: Vdc_m=global, Vdc_ref=global, rpm=global, rpm_ref=global
  wires:
  w_sens/1 -> Rate Transition1/1
  Hall/1 -> Rate Transition4/1
  RPMReq/1 -> Rate Transition6/1
  Rate Transition6/1 -> [rpm_ref], Sum/1
  Rate Transition1/1 -> rad/s->rpm/1
  rad/s->rpm/1 -> [rpm], Sum/2
  Sum/1 -> Speed controller/1
  Speed controller/1 -> Sum1/1, [Vdc_ref]
  Constant/1 -> Speed controller/2
  Rate Transition4/1 -> Commutation/1(Hall)
  Commutation/1(S) -> Rate Transition3/1
  Vdc/1 -> Rate Transition2/1
  Sum1/1 -> Voltage controller/1
  Constant1/1 -> Voltage controller/2
  Rate Transition2/1 -> Vdc filter/1
  Vdc filter/1 -> [Vdc_m], Sum1/2
  Rate Transition3/1 -> S/1
  Voltage controller/1 -> Duty/1

== system PMSM_FOC_Traction/PMSM/Resolver/Meas Vxy ==
  Electrical Reference{1..4} (4 alike) : fl_lib/Electrical/Electrical Elements/Electrical Reference
  PS-Simulink Converter : nesl_utility/PS-Simulink Converter  PhysicalDomain=network_engine_domain  SubClassName=ps_output  LeftPortType=input  RightPortType=output  PseudoPeriodic=off  Frequencies=[]  Unit=1  AffineConversion=off
  PS-Simulink Converter1 : nesl_utility/PS-Simulink Converter  PhysicalDomain=network_engine_domain  SubClassName=ps_output  LeftPortType=input  RightPortType=output  PseudoPeriodic=off  Frequencies=[]  Unit=1  AffineConversion=off
  Resistor : fl_lib/Electrical/Electrical Elements/Resistor  R=1e3 Ohm  i_specify=off  i_priority=None  i=0 A  i_nominal_specify=off  i_nominal_unit=A  i_nominal_value=1  v_specify=off  v_priority=None  v=0 V  v_nominal_specify=off  v_nominal_unit=V  v_nominal_value=1
  Resistor1 : fl_lib/Electrical/Electrical Elements/Resistor  R=1e3 Ohm  i_specify=off  i_priority=None  i=0 A  i_nominal_specify=off  i_nominal_unit=A  i_nominal_value=1  v_specify=off  v_priority=None  v=0 V  v_nominal_specify=off  v_nominal_unit=V  v_nominal_value=1
  VS1 : fl_lib/Electrical/Electrical Sensors/Voltage Sensor
  VS2 : fl_lib/Electrical/Electrical Sensors/Voltage Sensor
  x1 : PMIOPort  Side=Left
  x2 : PMIOPort  Port=2  Side=Left
  y1 : PMIOPort  Port=3  Side=Left
  y2 : PMIOPort  Port=4  Side=Left
  Vx : Outport  VectorParamsAs1DForOutWhenUnconnected=off
  Vy : Outport  Port=2  VectorParamsAs1DForOutWhenUnconnected=off
  wires:
  PS-Simulink Converter1/1 -> Vy/1
  PS-Simulink Converter/1 -> Vx/1
  connections:
  VS1/RConn1 -- PS-Simulink Converter/LConn1
  Resistor/RConn1 -- x2/RConn1 -- Electrical Reference2/LConn1
  Electrical Reference1/LConn1 -- VS1/RConn2
  y2/RConn1 -- Electrical Reference4/LConn1 -- Resistor1/RConn1
  VS2/LConn1 -- y1/RConn1 -- Resistor1/LConn1
  Electrical Reference3/LConn1 -- VS2/RConn2
  VS2/RConn1 -- PS-Simulink Converter1/LConn1
  Resistor/LConn1 -- x1/RConn1 -- VS1/LConn1

== system PMSM_FOC_Traction/PMSM/Resolver/Vp ==
  Electrical Reference1 : fl_lib/Electrical/Electrical Elements/Electrical Reference
  PS-Simulink Converter2 : nesl_utility/PS-Simulink Converter  PhysicalDomain=network_engine_domain  SubClassName=ps_output  LeftPortType=input  RightPortType=output  PseudoPeriodic=off  Frequencies=[]  Unit=1  AffineConversion=off
  VS1 : fl_lib/Electrical/Electrical Sensors/Voltage Sensor
  Vp1 : fl_lib/Electrical/Electrical Sources/AC Voltage Source  amp=5 V  shift=0 rad  frequency=1e4 Hz  omega=0 rad/s
  p1 : PMIOPort  Side=Right
  p2 : PMIOPort  Port=2  Side=Right
  Vp : Outport  VectorParamsAs1DForOutWhenUnconnected=off
  wires:
  PS-Simulink Converter2/1 -> Vp/1
  connections:
  VS1/RConn1 -- PS-Simulink Converter2/LConn1
  Electrical Reference1/LConn1 -- p2/RConn1 -- VS1/RConn2 -- Vp1/RConn1
  VS1/LConn1 -- Vp1/LConn1 -- p1/RConn1

== system PMSM_FOC_Traction/PMSM/Resolver_SinCos/If Action Subsystem ==
  In1 : Inport
  Action Port : ActionPort  ActionPortLabel=if(u1 == 1)
  Out1 : Outport
  wires:
  In1/1 -> Out1/1

== system PMSM_FOC_Traction/PMSM/Resolver_SinCos/If Action Subsystem1 ==
  In1 : Inport
  Action Port : ActionPort  ActionPortLabel=else
  Gain : Gain  Gain=-1
  Out1 : Outport
  wires:
  In1/1 -> Gain/1
  Gain/1 -> Out1/1

== system PMSM_FOC_Traction/PMSM/Resolver_SinCos/If Action Subsystem2 ==
  In1 : Inport
  Action Port : ActionPort  ActionPortLabel=if(u1 == 1)
  Out1 : Outport
  wires:
  In1/1 -> Out1/1

== system PMSM_FOC_Traction/PMSM/Resolver_SinCos/If Action Subsystem3 ==
  In1 : Inport
  Action Port : ActionPort  ActionPortLabel=else
  Gain : Gain  Gain=-1
  Out1 : Outport
  wires:
  In1/1 -> Gain/1
  Gain/1 -> Out1/1

== system PMSM_FOC_Traction/PMSM/Resolver_SinCos/Subsystem ==
  In1 : Inport
  Trigger : TriggerPort  VariantControl=Variant  SampleTimeType=periodic  SampleTime=-1  PortDimensions=1
  Out1 : Outport
  wires:
  In1/1 -> Out1/1

== system PMSM_FOC_Traction/PMSM/Resolver_SinCos/Subsystem1 ==
  In1 : Inport
  Trigger : TriggerPort  VariantControl=Variant  SampleTimeType=periodic  SampleTime=-1  PortDimensions=1
  Out1 : Outport
  wires:
  In1/1 -> Out1/1

== system PMSM_FOC_Traction/PMSM/Resolver_SinCos/Subsystem2 ==
  Trigger : TriggerPort  VariantControl=Variant  SampleTimeType=periodic  SampleTime=-1  PortDimensions=1
  Add : Sum
  Constant : Constant
  Constant1 : Constant  Value=2
  Memory : Memory  InheritSampleTime=on
  Mod : Math  Operator=mod  SaturateOnIntegerOverflow=on
  Out1 : Outport
  wires:
  Add/1 -> Mod/1, Memory/1
  Constant/1 -> Add/1
  Memory/1 -> Add/2
  Mod/1 -> Out1/1  "Theta"
  Constant1/1 -> Mod/2

== system PMSM_FOC_Traction/PMSM/Resolver_SinCos/Subsystem3 ==
  Trigger : TriggerPort  VariantControl=Variant  SampleTimeType=periodic  SampleTime=-1  PortDimensions=1
  Add : Sum
  Constant : Constant
  Constant1 : Constant  Value=2
  Memory : Memory  InheritSampleTime=on
  Mod : Math  Operator=mod  SaturateOnIntegerOverflow=on
  Out1 : Outport
  wires:
  Add/1 -> Mod/1, Memory/1
  Constant/1 -> Add/1
  Memory/1 -> Add/2
  Mod/1 -> Out1/1  "Theta"
  Constant1/1 -> Mod/2

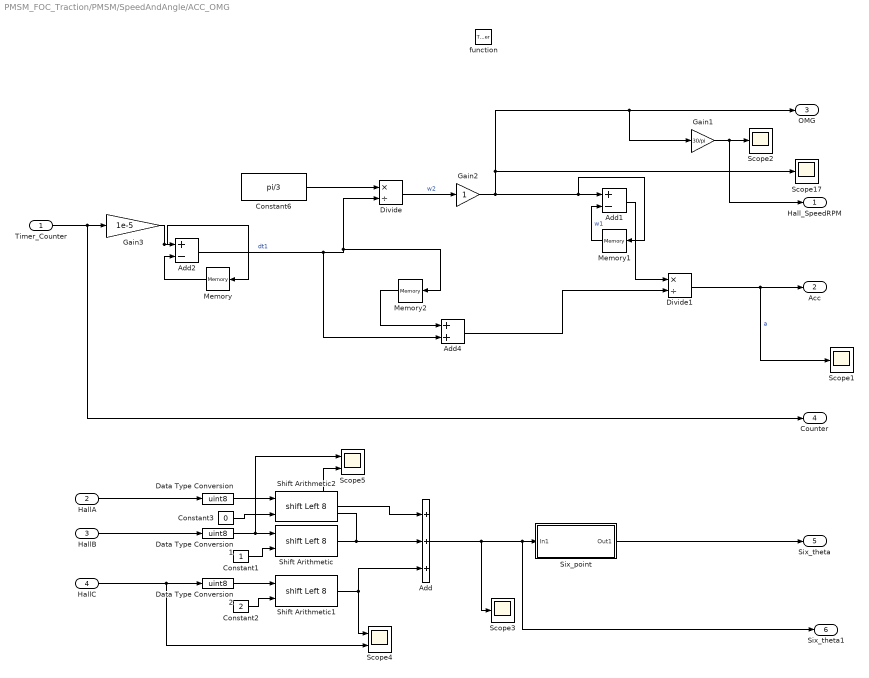
== system PMSM_FOC_Traction/PMSM/SpeedAndAngle/ACC_OMG ==
  Timer_Counter : Inport
  HallA : Inport  Port=2
  HallB : Inport  Port=3
  HallC : Inport  Port=4
  function : TriggerPort  TriggerType=either  VariantControl=Variant
  Add : Sum  Inputs=+++
  Add1 : Sum  Inputs=+-
  Add2 : Sum  Inputs=+-
  Add4 : Sum
  Constant1 : Constant  OutDataTypeStr=uint8
  Constant2 : Constant  Value=2  OutDataTypeStr=uint8
  Constant3 : Constant  Value=0  OutDataTypeStr=uint8
  Constant6 : Constant  Value=pi/3  OutDataTypeStr=single
  Data Type Conversion : DataTypeConversion  OutDataTypeStr=uint8
  Data Type Conversion1 : DataTypeConversion  OutDataTypeStr=uint8
  Data Type Conversion2 : DataTypeConversion  OutDataTypeStr=uint8
  Divide : Product  Inputs=*/
  Divide1 : Product  Inputs=*/
  Gain1 : Gain  Gain=30/pi  OutDataTypeStr=Inherit: Same as input  ParamDataTypeStr=Inherit: Same as input
  Gain2 : Gain  OutDataTypeStr=Inherit: Same as input  ParamDataTypeStr=Inherit: Same as input
  Gain3 : Gain  Gain=1e-5
  Memory : Memory  InheritSampleTime=on
  Memory1 : Memory  InheritSampleTime=on
  Memory2 : Memory  InheritSampleTime=on
  Scope{1..3,17} (4 alike) : Scope
  Scope4 : Scope  NumInputPorts=2
  Scope5 : Scope  NumInputPorts=2
  Shift Arithmetic : ArithShift  BitShiftNumberSource=Input port  BitShiftNumber=8  BitShiftDirection=Left
      settings: InputPortMap=u0,p1
  Shift Arithmetic1 : ArithShift  BitShiftNumberSource=Input port  BitShiftNumber=8  BitShiftDirection=Left
      settings: InputPortMap=u0,p1
  Shift Arithmetic2 : ArithShift  BitShiftNumberSource=Input port  BitShiftNumber=8  BitShiftDirection=Left
      settings: InputPortMap=u0,p1
  Six_point : Subsystem  TreatAsAtomicUnit=on
  Hall_SpeedRPM : Outport
  Acc : Outport  Port=2
  OMG : Outport  Port=3
  Counter : Outport  Port=4
  Six_theta : Outport  Port=5
  Six_theta1 : Outport  Port=6
  wires:
  Timer_Counter/1 -> Counter/1, Gain3/1
  Constant6/1 -> Divide/1
  Divide/1 -> Gain2/1  "w2"
  Memory/1 -> Add2/2
  Add2/1 -> Add4/2, Memory2/1, Divide/2  "dt1"
  Memory1/1 -> Add1/2  "w1"
  Add1/1 -> Divide1/1
  Add4/1 -> Divide1/2
  Divide1/1 -> Acc/1, Scope1/1  "a"
  Gain3/1 -> Memory/1, Add2/1
  Gain1/1 -> Hall_SpeedRPM/1, Scope2/1
  Memory2/1 -> Add4/1
  HallC/1 -> Scope4/2, Data Type Conversion2/1
  Data Type Conversion2/1 -> Shift Arithmetic1/1
  Constant2/1 -> Shift Arithmetic1/2
  Constant1/1 -> Shift Arithmetic/2
  Data Type Conversion1/1 -> Scope5/1, Shift Arithmetic/1
  HallA/1 -> Data Type Conversion/1
  Shift Arithmetic/1 -> Add/2, Scope5/2
  HallB/1 -> Data Type Conversion1/1
  Six_point/1(Out1) -> Six_theta/1
  Gain2/1 -> Gain1/1, OMG/1, Scope17/1, Memory1/1, Add1/1
  Shift Arithmetic1/1 -> Add/3, Scope4/1
  Add/1 -> Scope3/1, Six_theta1/1, Six_point/1(In1)
  Data Type Conversion/1 -> Shift Arithmetic2/1
  Shift Arithmetic2/1 -> Add/1
  Constant3/1 -> Shift Arithmetic2/2

== system PMSM_FOC_Traction/PMSM/SpeedAndAngle/ADC_IRQ ==
  Counter_ADC_IRQ : Inport
  Acc : Inport  Port=2
  OMG : Inport  Port=3
  Counter_Hall_IRQ : Inport  Port=4
  Six_theta : Inport  Port=5
  Add6 : Sum  Inputs=+-
  Add7 : Sum
  Gain2 : Gain  Gain=1e-5
  Gain3 : Gain  Gain=1e-5
  Gain4 : Gain  Gain=0.5
  Gain5 : Gain
  HallAngle_calibration : Subsystem
      settings: RTWSystemCode=Nonreusable function  RTWFcnNameOpts=Use subsystem name
  Math Function1 : Math  Operator=magnitude^2  SaturateOnIntegerOverflow=on
  Minus2 : Sum
  Product1 : Product
  Product2 : Product
  Hall_Angle : Outport
  wires:
  Gain5/1 -> Minus2/2
  Gain3/1 -> Math Function1/1
  Product2/1 -> Gain4/1
  Counter_Hall_IRQ/1 -> Add6/2
  Gain4/1 -> Minus2/1
  Add6/1 -> Gain3/1, Product1/2
  Math Function1/1 -> Product2/2
  Product1/1 -> Gain2/1
  Gain2/1 -> Gain5/1
  Counter_ADC_IRQ/1 -> Add6/1
  OMG/1 -> Product1/1
  Add7/1 -> HallAngle_calibration/1(Angle_input)
  Minus2/1 -> Add7/1
  Six_theta/1 -> Add7/2
  HallAngle_calibration/1(Angle_output) -> Hall_Angle/1  "SMO_Angle"
  Acc/1 -> Product2/1

== system PMSM_FOC_Traction/PMSM/W_R/Torque Sensor ==
  Ideal Torque Sensor : fl_lib/Mechanical/Mechanical Sensors/Ideal Torque Sensor
  PS-Simulink Converter : nesl_utility/PS-Simulink Converter  PhysicalDomain=network_engine_domain  SubClassName=ps_output  LeftPortType=input  RightPortType=output  PseudoPeriodic=off  Frequencies=[]  Unit=N*m  AffineConversion=off
  R : PMIOPort  Side=Right
  C : PMIOPort  Port=2  Side=Left
  tag scope: trqDynoOC=global
  wires:
  PS-Simulink Converter/1 -> [trqDynoOC]
  connections:
  PS-Simulink Converter/LConn1 -- Ideal Torque Sensor/RConn2
  R/RConn1 -- Ideal Torque Sensor/LConn1
  Ideal Torque Sensor/RConn1 -- C/RConn1

== system PMSM_FOC_Traction/Motor_Control/Motor_Control_Funtion/Angle_Speed_100us/Angle_Selector ==
  OPL_Theta : Inport
  CL_Theta : Inport  Port=2
  Motor_state : Inport  Port=3
  If1 : If  IfExpression=u1 ==2 | u1 ==3  ElseIfExpressions=u1 ==4  ShowElse=off
  Merge : Merge
  Scope : Scope  NumInputPorts=2
  Subsystem : Subsystem
  Subsystem1 : Subsystem
  Theta : Outport
  wires:
  Motor_state/1 -> If1/1
  If1/1 -> Subsystem/Action
  OPL_Theta/1 -> Scope/1, Subsystem/1(In1)
  CL_Theta/1 -> Scope/2, Subsystem1/1(In1)
  Subsystem/1(Out1) -> Merge/1
  Subsystem1/1(Out1) -> Merge/2
  Merge/1 -> Theta/1  "FOC_Angle"
  If1/2 -> Subsystem1/Action

== system PMSM_FOC_Traction/Motor_Control/Motor_Control_Funtion/Angle_Speed_100us/Flux_OBSERVER ==
  i_alpha : Inport  OutDataTypeStr=single
  i_beta : Inport  Port=2  OutDataTypeStr=single
  u_alpha : Inport  Port=3  OutDataTypeStr=single
  u_beta : Inport  Port=4  OutDataTypeStr=single
  Action Port : ActionPort  ActionPortLabel=if(u1==1)
  Abs : Abs  OutDataTypeStr=single
  Moving Average : dspstat3/Moving Average  Method=Exponential weighting  ForgettingFactorPort=off  SpecifyWindowLength=on  WindowLength=4  ForgettingFactor=0.99  SimulateUsing=Code generation
  equ3.12 : Subsystem
  equ3.6 : Subsystem
  equ3.9 : Subsystem
  sin_cos : Outport  OutDataTypeStr=single
  omega_e_hat : Outport  Port=2  OutDataTypeStr=single
  wires:
  i_beta/1 -> equ3.9/4(i_beta), equ3.6/3(i_beta)
  i_alpha/1 -> equ3.9/3(i_alpha), equ3.6/1(i_alpha)
  u_alpha/1 -> equ3.6/2(u_alpha)
  u_beta/1 -> equ3.6/4(u_beta)
  equ3.6/1(y1) -> equ3.9/1(y1)
  equ3.6/2(y2) -> equ3.9/2(y2)
  equ3.9/1(eta_x1_hat) -> equ3.12/1(eta_x1_hat)  "eta_x1"
  equ3.9/2(eta_x2_hat) -> equ3.12/2(eta_x2_hat)  "eta_x2"
  equ3.12/1(Theta) -> sin_cos/1
  Abs/1 -> Moving Average/1
  equ3.12/2(omega_e_hat) -> Abs/1, omega_e_hat/1
  Moving Average/1 -> equ3.9/5(omega_e_hat), equ3.6/5(omega_e_hat)

== system PMSM_FOC_Traction/Motor_Control/Motor_Control_Funtion/Angle_Speed_100us/HIGH_SMO ==
  Valpha : Inport
  Vbeta : Inport  Port=2
  Ialpha : Inport  Port=3
  Ibeta : Inport  Port=4
  Equ1 : Subsystem
  Equ2 : Subsystem
  Equ3 : Subsystem
  Equ4 : Subsystem
  QPLL : Subsystem
  Sign : Signum
  Sign1 : Signum
  Sum2 : Sum  Inputs=|+-
  Sum6 : Sum  Inputs=|+-
  sin_cos : Outport
  omega_hat : Outport  Port=2
  wires:
  Sum6/1 -> Sign1/1
  Sum2/1 -> Sign/1
  Sign/1 -> Equ3/3(alpha_err), Equ1/5(alpha_err)  "alphaErr"
  Ialpha/1 -> Sum2/2
  Sign1/1 -> Equ4/3(beta_err), Equ2/5(beta_err)  "betaErr"
  Ibeta/1 -> Sum6/2
  Equ1/1(i_alpha_hat) -> [i_alpha_hat]
  [e_alpha_hat] -> Equ1/2(e_alpha_hat)
  Valpha/1 -> Equ1/3(u_alpha)
  [e_beta_hat] -> Equ2/3(e_beta_hat)
  Vbeta/1 -> Equ2/4(u_beta)
  Equ2/1(i_beta_hat) -> [i_beta_hat]
  [i_beta_hat] -> Equ1/4(I_beta_hat)
  [i_beta_hat] -> Sum6/1
  [i_alpha_hat] -> Sum2/1
  [i_alpha_hat] -> Equ2/2(i_alpha_hat)
  [omega_hat] -> Equ3/1(omega_hat)
  [e_beta_hat] -> Equ3/2(e_beta_hat)
  [omega_hat] -> Equ4/1(omega_hat)
  [e_alpha_hat] -> Equ4/2(e_alpha_hat)
  [omega_hat] -> Equ1/1(omega_hat)
  Equ4/1(e_beta_hat) -> [e_beta_hat]  "e_beta_hat"
  Equ3/1(e_alpha_hat) -> [e_alpha_hat]  "e_alpha_hat"
  [e_alpha_hat] -> QPLL/1(e_alpha_hat)
  [e_beta_hat] -> QPLL/2(e_beta_hat)
  QPLL/2(speed_hat) -> [omega_hat], omega_hat/1
  QPLL/1(sin_cos) -> sin_cos/1  "sin_cos"
  [omega_hat] -> Equ2/1(omega_hat)

== system PMSM_FOC_Traction/Motor_Control/Motor_Control_Funtion/Angle_Speed_100us/Resolver_Observer ==
  Resolver_SinCos : Inport
  Action Port : ActionPort  ActionPortLabel=if(u1==1)
  Angle_calibration : Subsystem  TreatAsAtomicUnit=on
      settings: RTWSystemCode=Nonreusable function  RTWFcnNameOpts=Use subsystem name
  Resolver_Angle_cacl : Subsystem  TreatAsAtomicUnit=on
      settings: RTWSystemCode=Nonreusable function  RTWFcnNameOpts=Use subsystem name  RTWFileNameOpts=Use subsystem name  FunctionInterfaceSpec=Allow arguments (Optimized)
  Scope : Scope
  Scope1 : Scope
  Obser_Speed : Outport
  Obser_Theta : Outport  Port=2
  wires:
  Resolver_Angle_cacl/1(Velocity) -> Scope/1, Obser_Speed/1  "Obser_Speed"
  Resolver_Angle_cacl/2(Angle) -> Angle_calibration/1(Angle_input)
  Resolver_SinCos/1 -> Resolver_Angle_cacl/1(Sin_Cos)
  Angle_calibration/1(Angle_output) -> Scope1/1, Obser_Theta/1  "Obser_Angle"
